simulink model "sysp7_LA"  (R2023a)
settings: Solver=ode15s  StartTime=0.0  StopTime=30  MaxStep=1E-3  RelTol=1E-3
settings Model: Creator=Ariel  LastModifiedBy=Ariel
settings DataIOCC: ReturnWorkspaceOutputs=off  TimeSaveName=t
settings DebuggingCC: AlgebraicLoopMsg=none  ArtificialAlgebraicLoopMsg=none  MaxConsecutiveZCsMsg=none  ModelReferenceExtraNoncontSigs=none  OperatingPointInterfaceChecksumMismatchMsg=none

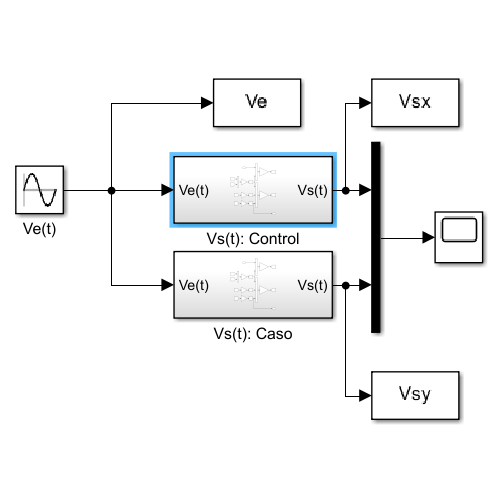
[thumbnail: Simulink's stored preview of the top-level diagram]
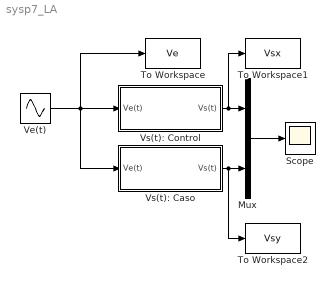
== system sysp7_LA ==
  Mux : Mux  Inputs=2
  Scope : Scope
  To Workspace : ToWorkspace  VariableName=Ve  SaveFormat=Timeseries  SampleTime=-1
  To Workspace1 : ToWorkspace  VariableName=Vsx  SaveFormat=Timeseries  SampleTime=-1
  To Workspace2 : ToWorkspace  VariableName=Vsy  SaveFormat=Timeseries  SampleTime=-1
  Ve(t) : Sin  Frequency=pi/2  SampleTime=0
  Vs(t): Caso : Subsystem
  Vs(t): Control : Subsystem
  wires:
  Mux/1 -> Scope/1
  Vs(t): Control/1(Vs(t)) -> To Workspace1/1, Mux/1
  Vs(t): Caso/1(Vs(t)) -> To Workspace2/1, Mux/2
  Ve(t)/1 -> Vs(t): Control/1(Ve(t)), Vs(t): Caso/1(Ve(t)), To Workspace/1

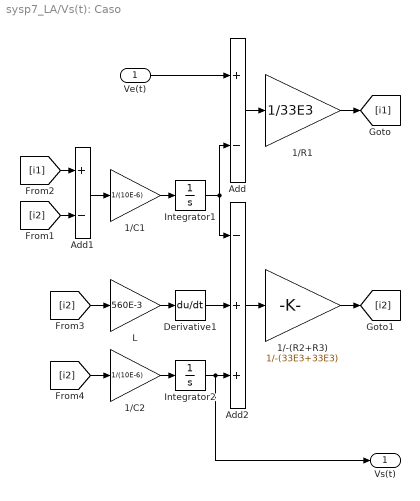
== system sysp7_LA/Vs(t): Caso ==
  Ve(t) : Inport
  1/-(R2+R3) : Gain  Gain=1/-(33E3+33E3)
  1/C1 : Gain  Gain=1/(10E-6)
  1/C2 : Gain  Gain=1/(10E-6)
  1/R1 : Gain  Gain=1/33E3
  Add : Sum  Inputs=+-
  Add1 : Sum  Inputs=+-
  Add2 : Sum  Inputs=-++
  Derivative1 : Derivative
  Integrator1 : Integrator
  Integrator2 : Integrator
  L : Gain  Gain=560E-3
  Vs(t) : Outport
  wires:
  Ve(t)/1 -> Add/1
  Add1/1 -> 1/C1/1
  [i1] -> Add1/1
  [i2] -> Add1/2
  Add/1 -> 1/R1/1
  1/R1/1 -> [i1]
  Integrator1/1 -> Add/2, Add2/1
  1/C1/1 -> Integrator1/1
  [i2] -> L/1
  L/1 -> Derivative1/1
  1/C2/1 -> Integrator2/1
  [i2] -> 1/C2/1
  Integrator2/1 -> Vs(t)/1, Add2/3
  Derivative1/1 -> Add2/2
  Add2/1 -> 1/-(R2+R3)/1
  1/-(R2+R3)/1 -> [i2]

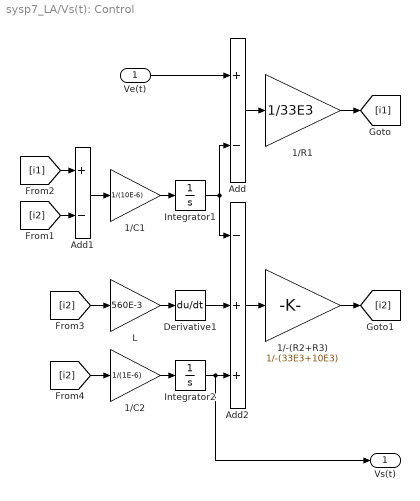
== system sysp7_LA/Vs(t): Control ==
  Ve(t) : Inport
  1/-(R2+R3) : Gain  Gain=1/-(33E3+10E3)
  1/C1 : Gain  Gain=1/(10E-6)
  1/C2 : Gain  Gain=1/(1E-6)
  1/R1 : Gain  Gain=1/33E3
  Add : Sum  Inputs=+-
  Add1 : Sum  Inputs=+-
  Add2 : Sum  Inputs=-++
  Derivative1 : Derivative
  Integrator1 : Integrator
  Integrator2 : Integrator
  L : Gain  Gain=560E-3
  Vs(t) : Outport
  wires:
  Ve(t)/1 -> Add/1
  Add1/1 -> 1/C1/1
  [i1] -> Add1/1
  [i2] -> Add1/2
  Add/1 -> 1/R1/1
  1/R1/1 -> [i1]
  Integrator1/1 -> Add/2, Add2/1
  1/C1/1 -> Integrator1/1
  [i2] -> L/1
  L/1 -> Derivative1/1
  1/C2/1 -> Integrator2/1
  [i2] -> 1/C2/1
  Integrator2/1 -> Vs(t)/1, Add2/3
  Derivative1/1 -> Add2/2
  Add2/1 -> 1/-(R2+R3)/1
  1/-(R2+R3)/1 -> [i2]
